simulink model "PWM_controller_interface"  (R2014b)
settings: Solver=FixedStepDiscrete  StartTime=0.0  StopTime=inf  RelTol=1e-3
undefined symbols (not defined in the file): AXI4, Lite
libraries: axiinterfacelib x3, simulink x1
settings Model: FPTRunName=FPA_Reference  SimulationMode=external  Creator=variable  LastModifiedBy=maclab3
settings SolverCC: PositivePriorityOrder=on
settings DataIOCC: SaveOutput=off  SaveTime=off
settings OptimizationCC: OptimizeModelRefInitCode=on  LifeSpan=1  MaxStackSize=64
settings DebuggingCC: UnderspecifiedInitializationDetection=Classic  MergeDetectMultiDrivingBlocksExec=none
settings HardwareCC: ProdLargestAtomicInteger=Long  ProdLargestAtomicFloat=Double  ProdEndianess=LittleEndian  ProdHWDeviceType=ARM Compatible->ARM Cortex  TargetLargestAtomicInteger=Long  TargetLargestAtomicFloat=Double  TargetIntDivRoundTo=Zero  TargetEndianess=LittleEndian  TargetHWDeviceType=ARMCortex  ProdEqTarget=off
settings RTWCC: SystemTargetFile=ert.tlc  TLCOptions=-aInlineSetEventsForThisBaseRateFcn=TLC_FALSE -aSuppressMultiTaskScheduler=TLC_FALSE  TemplateMakefile=ert_default_tmf  Description=Embedded Coder  ProcessScript=idelink_ert_make_rtw_hook  Toolchain=Xilinx Software Development Kit (SDK) 2013.4
settings CodeAppCC: IgnoreCustomStorageClasses=off
settings ERTTargetCC: ParMdlRefBuildCompliant=off  GeneratePreprocessorConditionals=Disable all  CPPClassGenCompliant=off

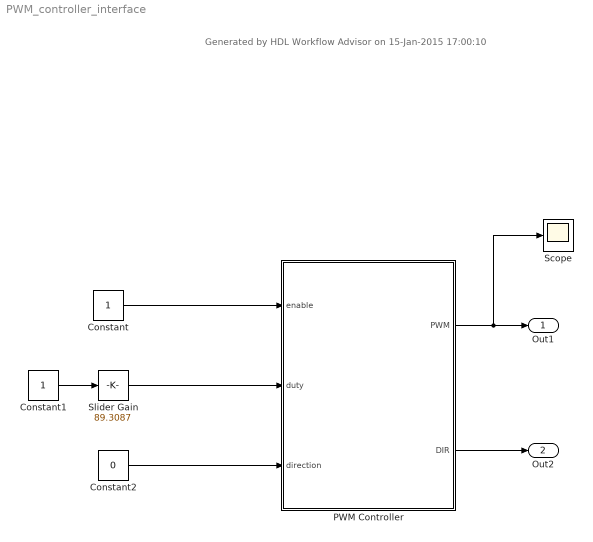
== system PWM_controller_interface ==
  note: Generated by HDL Workflow Advisor on 15-Jan-2015 17:00:10
  Constant : Constant  OutDataTypeStr=boolean  SampleTime=1
  Constant1 : Constant  OutDataTypeStr=uint8  SampleTime=1
  Constant2 : Constant  Value=0  OutDataTypeStr=boolean  SampleTime=1
  PWM Controller : Subsystem  TreatAsAtomicUnit=on  SystemSampleTime=1  mask(AXI4-Lite/AXI4 Interface){}
      mask help:
      | This is an automatically generated subsystem block.
      | This contains the AXI4-Lite/AXI4 interface which communicates with the PWM_controller_PWM_Controller_ipcore IPCore generated from PWM_controller/PWM Controller subsystem.
      mask Display: disp(sprintf('Xilinx Zynq \nAXI4-Lite/AXI4 Interface'));
  Scope : Scope
  Slider Gain : simulink/Math Operations/Slider Gain  low=0  gain=89.3087  high=255
  Out1 : Outport
  Out2 : Outport  Port=2
  wires:
  PWM Controller/2(DIR) -> Out2/1
  PWM Controller/1(PWM) -> Out1/1, Scope/1
  Slider Gain/1 -> PWM Controller/2(duty)
  Constant2/1 -> PWM Controller/3(direction)
  Constant1/1 -> Slider Gain/1
  Constant/1 -> PWM Controller/1(enable)

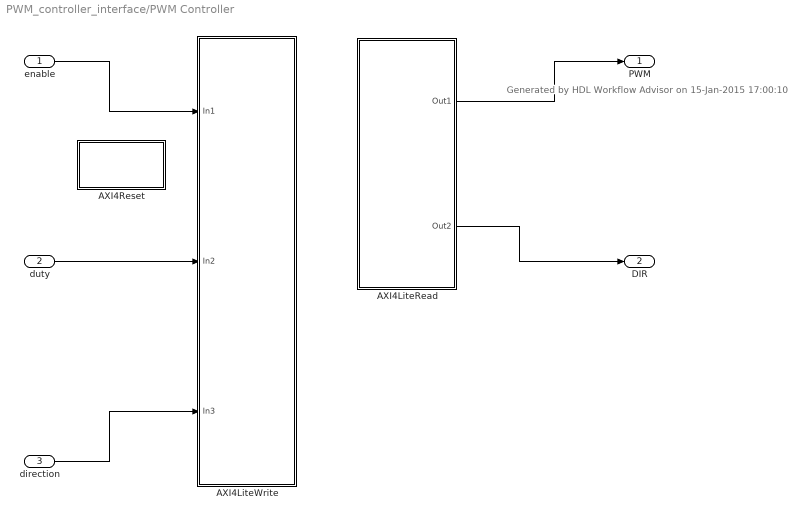
== system PWM_controller_interface/PWM Controller ==
  note: Generated by HDL Workflow Advisor on 15-Jan-2015 17:00:10
  enable : Inport
  duty : Inport  Port=2  OutDataTypeStr=fixdt(0,8,0)
  direction : Inport  Port=3
  AXI4LiteRead : Subsystem  Priority=10
  AXI4LiteWrite : Subsystem  Priority=1
  AXI4Reset : Subsystem  mask(System Initialize){ShowInLibBrowser=0}
      mask prompts: ShowInLibBrowser "Simulink:masks:CustCodeMaskParam1_MP"
      settings: CopyFcn=cccopyfcn(gcb)  OpenFcn=ccopenfcn('System Initialize Function')
      mask Help: eval('feval(''rtwprivate'',''rtwhelpview'',''rtw_sys_initialize_block'')');
      mask Display: disp('System\nInitialize');
  PWM : Outport
  DIR : Outport  Port=2
  wires:
  enable/1 -> AXI4LiteWrite/1(In1)
  duty/1 -> AXI4LiteWrite/2(In2)
  direction/1 -> AXI4LiteWrite/3(In3)
  AXI4LiteRead/1(Out1) -> PWM/1
  AXI4LiteRead/2(Out2) -> DIR/1

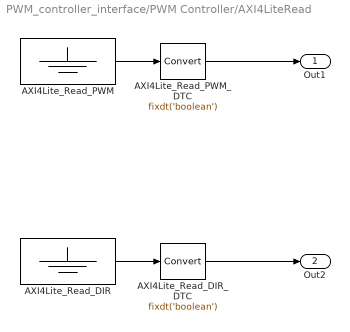
== system PWM_controller_interface/PWM Controller/AXI4LiteRead ==
  AXI4Lite_Read_DIR : Ground
  AXI4Lite_Read_DIR_DTC : DataTypeConversion  OutDataTypeStr=fixdt('boolean')  ConvertRealWorld=Stored Integer (SI)
  AXI4Lite_Read_PWM : Ground
  AXI4Lite_Read_PWM_DTC : DataTypeConversion  OutDataTypeStr=fixdt('boolean')  ConvertRealWorld=Stored Integer (SI)
  Out1 : Outport
  Out2 : Outport  Port=2
  wires:
  AXI4Lite_Read_PWM/1 -> AXI4Lite_Read_PWM_DTC/1
  AXI4Lite_Read_PWM_DTC/1 -> Out1/1
  AXI4Lite_Read_DIR_DTC/1 -> Out2/1
  AXI4Lite_Read_DIR/1 -> AXI4Lite_Read_DIR_DTC/1

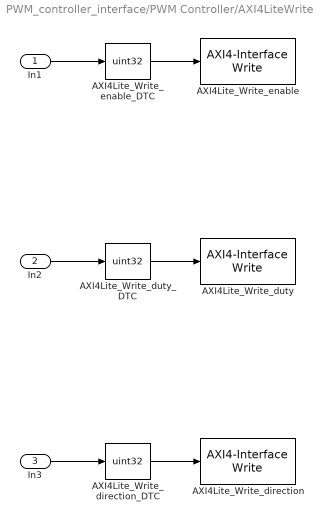
== system PWM_controller_interface/PWM Controller/AXI4LiteWrite ==
  In1 : Inport
  In2 : Inport  Port=2
  In3 : Inport  Port=3
  AXI4Lite_Write_direction : axiinterfacelib/AXI4-Interface Write  Priority=3  AXIInterfaceType=AXI4-Lite  DeviceName=/dev/mwipcore  RegisterOffset=hex2dec('108')  blockPlatform=ZYNQ  SimulateUsing=Interpreted execution
  AXI4Lite_Write_direction_DTC : DataTypeConversion  OutDataTypeStr=uint32  ConvertRealWorld=Stored Integer (SI)
  AXI4Lite_Write_duty : axiinterfacelib/AXI4-Interface Write  Priority=2  AXIInterfaceType=AXI4-Lite  DeviceName=/dev/mwipcore  RegisterOffset=hex2dec('104')  blockPlatform=ZYNQ  SimulateUsing=Interpreted execution
  AXI4Lite_Write_duty_DTC : DataTypeConversion  OutDataTypeStr=uint32  ConvertRealWorld=Stored Integer (SI)
  AXI4Lite_Write_enable : axiinterfacelib/AXI4-Interface Write  Priority=1  AXIInterfaceType=AXI4-Lite  DeviceName=/dev/mwipcore  RegisterOffset=hex2dec('100')  blockPlatform=ZYNQ  SimulateUsing=Interpreted execution
  AXI4Lite_Write_enable_DTC : DataTypeConversion  OutDataTypeStr=uint32  ConvertRealWorld=Stored Integer (SI)
  wires:
  In1/1 -> AXI4Lite_Write_enable_DTC/1
  AXI4Lite_Write_enable_DTC/1 -> AXI4Lite_Write_enable/1
  In2/1 -> AXI4Lite_Write_duty_DTC/1
  AXI4Lite_Write_duty_DTC/1 -> AXI4Lite_Write_duty/1
  AXI4Lite_Write_direction_DTC/1 -> AXI4Lite_Write_direction/1
  In3/1 -> AXI4Lite_Write_direction_DTC/1

== system PWM_controller_interface/PWM Controller/AXI4Reset ==
